simulink model "LQR_2018"  (R2018b)
settings: Solver=VariableStepAuto  StartTime=0.0  StopTime=40.0  RelTol=1e-3
values from neighbouring files (symbols this model uses):
  beta = params(1)    [model.m]
  g = 9.8105    [model.m]    (also in weryfikacja.m)
  I = 0.0226    [model.m]    (also in weryfikacja.m = 0.029572173408)
  K = params(3)    [model.m]
  K_lqr = lqr(A,B,Q,R)    [weryfikacja.m]
  tau = params(4)    [model.m]
  U = params(2)    [model.m]
  xep = [deg2rad(-2*21.37) 0 2000]    [weryfikacja.m]
settings Model: Creator=turgo  LastModifiedBy=turgo
settings DataIOCC: ReturnWorkspaceOutputs=on
settings DebuggingCC: UnconnectedInputMsg=none  UnconnectedOutputMsg=none  UnconnectedLineMsg=none  SFMachineParentedDataDiag=error

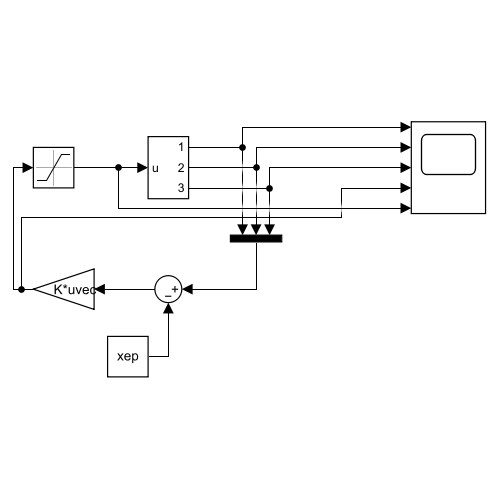
[thumbnail: Simulink's stored preview of the top-level diagram]
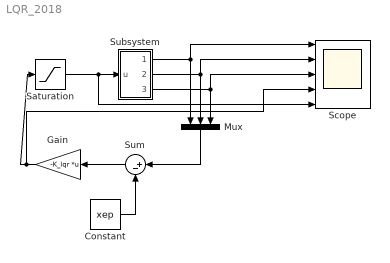
== system LQR_2018 ==
  Constant : Constant  Value=xep  VectorParams1D=off
  Gain : Gain  Gain=-K_lqr  Multiplication=Matrix(K*u) (u vector)
  Mux : Mux  Inputs=3
  Saturation : Saturate  UpperLimit=1  LowerLimit=-1
  Scope : Scope  NumInputPorts=5
  Subsystem : Subsystem
  Sum : Sum  Inputs=|+-
  wires:
  Subsystem/1(Out1) -> Scope/1, Mux/1
  Subsystem/2(Out2) -> Mux/2, Scope/2
  Subsystem/3(Out3) -> Mux/3, Scope/3
  Constant/1 -> Sum/2
  Sum/1 -> Gain/1
  Mux/1 -> Sum/1
  Saturation/1 -> Scope/5, Subsystem/1(u)
  Gain/1 -> Scope/4, Saturation/1

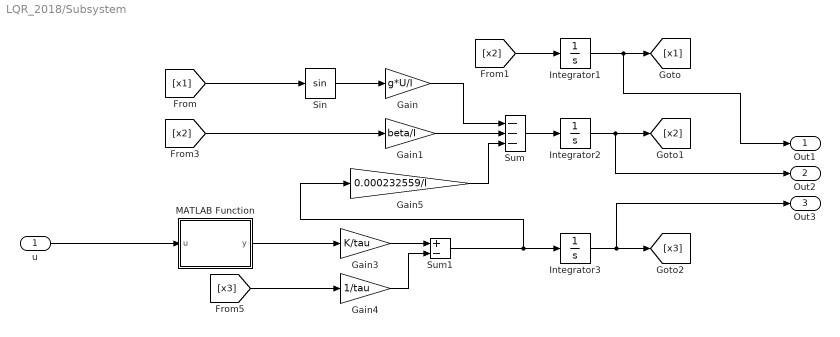
== system LQR_2018/Subsystem ==
  u : Inport
  Gain : Gain  Gain=g*U/I
  Gain1 : Gain  Gain=beta/I
  Gain3 : Gain  Gain=K/tau
  Gain4 : Gain  Gain=1/tau
  Gain5 : Gain  Gain=0.000232559/I
  Integrator1 : Integrator  InitialCondition=3
  Integrator2 : Integrator  InitialCondition=0.2
  Integrator3 : Integrator
  MATLAB Function : MATLAB Function  TreatAsAtomicUnit=on
  Sin : Trigonometry
  Sum : Sum  Inputs=---
  Sum1 : Sum  Inputs=+-
  Out1 : Outport
  Out2 : Outport  Port=2
  Out3 : Outport  Port=3
  wires:
  [x1] -> Sin/1
  Integrator1/1 -> Out1/1, [x1]
  Sum/1 -> Integrator2/1
  Sin/1 -> Gain/1
  Gain/1 -> Sum/1
  Gain5/1 -> Sum/3
  Gain4/1 -> Sum1/2
  Gain3/1 -> Sum1/1
  [x2] -> Gain1/1
  [x2] -> Integrator1/1
  Integrator3/1 -> Out3/1, [x3]
  Gain1/1 -> Sum/2
  Integrator2/1 -> Out2/1, [x2]
  u/1 -> MATLAB Function/1(u)
  Sum1/1 -> Gain5/1, Integrator3/1
  MATLAB Function/1(y) -> Gain3/1
  [x3] -> Gain4/1

== matlab function LQR_2018/Subsystem/MATLAB Function ==
  data: u input; y output
function y = fcn(u)

y = 211.6*u + 0.953;
